simulink model "raspi_websocket_cam"  (Simulink 10.0)
settings: Solver=FixedStepDiscrete  StartTime=0.0  StopTime=Inf  RelTol=1e-3  EnableMultiTasking=on
libraries: raspberrypiAVlib x1, raspberrypiNetworklib x1
settings Model: FPTRunName=Active  Creator=The MathWorks, Inc.  LastModifiedBy=kkoichi  EnablePacing=on  ExtModeTrigDuration=2
settings SolverCC: PositivePriorityOrder=on
settings DataIOCC: LimitDataPoints=on  SaveOutput=off  SignalLogging=off  DSMLogging=off  SaveTime=off
settings OptimizationCC: ExpressionDepthLimit=2147483647  LifeSpan=Inf  MaxStackSize=64
settings DebuggingCC: SaveWithDisabledLinksMsg=none  SaveWithParameterizedLinksMsg=none  FcnCallInpInsideContextMsg=warning  AllowSymbolicDim=off  StateNameClashWarn=warning
settings HardwareCC: ProdLargestAtomicInteger=Long  ProdLargestAtomicFloat=Double  ProdIntDivRoundTo=Zero  ProdEndianess=LittleEndian  ProdLongLongMode=on  ProdHWDeviceType=ARM Compatible->ARM Cortex  UseEmbeddedCoderFeatures=off  UseSimulinkCoderFeatures=off
settings RTWCC: Description=Embedded Coder  SystemTargetFile=ert.tlc  HardwareBoard=Raspberry Pi  TLCOptions="-aInlineSetEventsForThisBaseRateFcn=TLC_FALSE -aSuppressMultiTaskScheduler=TLC_FALSE  -aRateBasedStepFcn=0"  TemplateMakefile=ert_default_tmf  GenerateReport=on  RTWVerbose=off  Toolchain=GNU GCC Embedded Linux  BuildConfiguration=Faster Runs  LaunchReport=on
settings MATStruct: className=codertarget.tools.BuildHook  argsTopModelOnly=[]  excludedModels=[]  includeReferencedModels=on  includeTopModel=on  enabled=on  UseCoderTarget=[1.0]  TargetHardware=Raspberry Pi  RTOS=Linux  RTOSBaseRateTaskPriority=40  DetectTaskOverruns=[0.0]  Scheduler_interrupt_source=[0.0]  DataVersion=2016.02  IOBlocksMode=deployed  IPAddress=codertarget.raspi.getDeviceAddress  Port=17725  Verbose=[0.0]  RunInBackground=[0.0]  Configuration=XCP on TCP/IP  signalBufferSize=[1000000.0]  DeviceAddress=192.168.1.107  Username=pi  Password=raspberry  BuildDir=/home/pi  SerialNumber=172.19.74.109  OnlineBuildDir=/home/pi  BuildAction=Build and run  RunOnBoot=[0.0]  SPI0CE0BusSpeed=500  SPI0CE1BusSpeed=500  CANBusSpeed=500  CANOscillatorFrequency=16  InterruptPin=12  AllowAllFilter=[1.0]  Buffer0IDType=Normal  AcceptanceMask0=0  AcceptanceFilter0=255  AcceptanceFilter1=255  Buffer1IDType=Normal  AcceptanceMask1=0  AcceptanceFilter2=255  AcceptanceFilter3=255  AcceptanceFilter4=255  AcceptanceFilter5=255  InverseFilter0=[0.0]  InverseFilter1=[0.0]  Buffer2IDType=Extended  AcceptanceMask2=0  InverseFilter2=[0.0]  Buffer3IDType=Extended  AcceptanceMask3=0  InverseFilter3=[0.0]  BrokerAddress=mqtt.thingspeak.com  TransportLayerType=TCP/IP  ModelTransportDataFcn=codertarget.raspi.ioclient.getModelTransportInfo  ServerDeployFcn=codertarget.raspi.ioclient.deployServer  TransportLayerTypeOnline=Internet  Modbus_comms=TCP/IP  Modbus_mode=Master  Modbus_serverRemotePort=502  Modbus_serverLocalPort=502  Modbus_configCoil=1  Modbus_CoilAddr=0  Modbus_CoilNum=1  Modbus_configInput=1  Modbus_InputAddr=0  Modbus_InputNum=1  Modbus_configHoldingReg=1  Modbus_HoldingRegAddr=0  Modbus_HoldingRegNum=1  Modbus_configInputReg=1  Modbus_InputRegAddr=0  Modbus_InputRegNum=1  Modbus_MasterTimeout=100  EnableDeployment=[0.0]  IPAddressType=Device address  WebSocketPort=8000  HTTPPort=8888
settings CodeAppCC: ForceParamTrailComments=on  OperatorAnnotations=on  MangleLength=10  MATLABSourceComments=on
settings ERTTargetCC: MultiwordLength=2048  ERTCustomFileBanners=off  SupportContinuousTime=on  SupportNonInlinedSFcns=on  RemoveResetFunc=off  SupportVariableSizeSignals=on  ModelStepFunctionPrototypeControlCompliant=off  ExtModeTransport=2  ExtModeStaticAlloc=on  ExtModeMexFile=ext_xcp  ExtModeIntrfLevel=Level2 - Open
settings ConfigComp: CovExternalEMLEnable=off  CovSFcnEnable=off

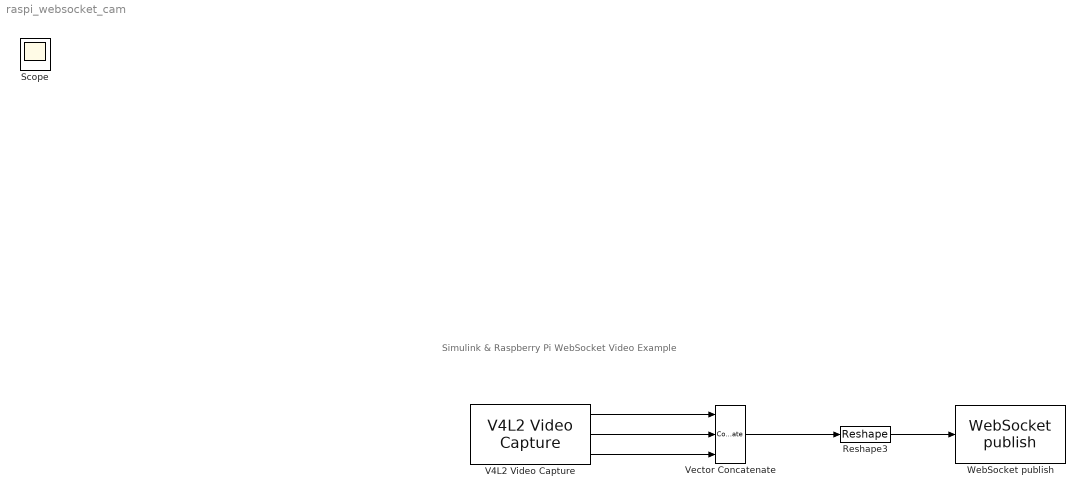
== system raspi_websocket_cam ==
  note: Simulink & Raspberry Pi WebSocket Video Example
  Reshape3 : Reshape
  V4L2 Video Capture : raspberrypiAVlib/V4L2 Video Capture  DeviceName=/dev/video0  Resolution=160x120  CustomResolution=[160,120]  PixelFormat=RGB  SampleTime=0.1  pixelOrder=Planar  simOutput=Colorbars  imSizeSelection=320x240  imSize=[640, 480]  roi=[0, 0, 640, 480]  m_devName='/dev/video0'  blockPlatform=Raspberry Pi
      settings: SourceProductBaseCode=RASPPI
      settings: AttributesFormatString=|
      | <DeviceName=%<DeviceName>>
      | <imSizeSelection=%<imSizeSelection>>
      | <PixelFormat=%<PixelFormat>>
      | <SampleTime=%<SampleTime>>
  Vector Concatenate : Concatenate  NumInputs=3  Mode=Multidimensional array  ConcatenateDimension=3
  WebSocket publish : raspberrypiNetworklib/WebSocket publish  UniqueBlockID=CameraData  IPAddress=192.168.1.107  Port=9137  NumberOfSignals=1  webSocketId=raspi_websocket_cam/WebSocket_publish  BlockPlatform=RASPBERRYPI
      settings: SourceProductBaseCode=RASPPI
      settings: AttributesFormatString=|
      | <IPAddress=%<IPAddress>>
      | <Port=%<Port>>
  Scope : Scope
  wires:
  V4L2 Video Capture/1 -> Vector Concatenate/1
  V4L2 Video Capture/2 -> Vector Concatenate/2
  V4L2 Video Capture/3 -> Vector Concatenate/3
  Reshape3/1 -> WebSocket publish/1
  Vector Concatenate/1 -> Reshape3/1
